simulink model "RecurDyn_Host_Block_23_2"  (R2024a)
settings: Solver=ode45  StartTime=0.0  StopTime=1.0  FixedStep=Control_timestep  RelTol=1e-3  AbsTol=1e-6
values from neighbouring files (symbols this model uses):
  GCoSim_Name = 'GCoSim1'    [car_ver1_GCoSim1.m]    (also in car_ver1_GCoSim2.m = 'GCoSim2'; pure_GCoSim1.m)
  GCoSim_Name_n = r_temp___(2)    [car_ver1_GCoSim1.m]    (also in car_ver1_GCoSim2.m; pure_GCoSim1.m)
  Matlab_version = str2double(splited_Version__(1))    [car_ver1_GCoSim1.m]    (also in car_ver1_GCoSim2.m; pure_GCoSim1.m)
  Output_File = 'car_ver1_GCoSim1_GCoSim1'    [car_ver1_GCoSim1.m]    (also in car_ver1_GCoSim2.m = 'car_ver1_GCoSimulink_GCoSim2'; pure_GCoSim1.m = 'pure_GCoSim1')
  Output_file_n = r_temp___(2)    [car_ver1_GCoSim1.m]    (also in car_ver1_GCoSim2.m; pure_GCoSim1.m)
  Plant_inputs_num = r_temp___(1)    [car_ver1_GCoSim1.m]    (also in car_ver1_GCoSim2.m; pure_GCoSim1.m)
  Plant_outputs_num = r_temp___(1)    [car_ver1_GCoSim1.m]    (also in car_ver1_GCoSim2.m; pure_GCoSim1.m)
  RecurDyn = 'C:\Program Files\FunctionBay, Inc\RecurDyn 2024\Bin\'    [car_ver1_GCoSim1.m]    (also in car_ver1_GCoSim2.m; pure_GCoSim1.m)
  RecurDyn_controltimestep = 1.e-003    (= 0.001)    [car_ver1_GCoSim1.m]    (also in car_ver1_GCoSim2.m; pure_GCoSim1.m)
  RecurDyn_model = 'car_ver1.rdyn'    [car_ver1_GCoSim1.m]    (also in car_ver1_GCoSim2.m; pure_GCoSim1.m = 'pure.rdyn')
  RecurDyn_model_n = r_temp___(2)    [car_ver1_GCoSim1.m]    (also in car_ver1_GCoSim2.m; pure_GCoSim1.m)
settings Model: Creator=hgildong  LastModifiedBy=Dell
settings SolverCC: AutoScaleAbsTol=off  AlgebraicLoopSolver=TrustRegion
settings DataIOCC: SaveFormat=Array  SignalLoggingSaveFormat=ModelDataLogs  ReturnWorkspaceOutputs=off
settings OptimizationCC: BooleanDataType=off  ExpressionDepthLimit=2147483647  InitFltsAndDblsToZero=on  LifeSpan=inf
settings DebuggingCC: SaveWithParameterizedLinksMsg=none  UnderspecifiedInitializationDetection=Classic  MergeDetectMultiDrivingBlocksExec=none  SignalResolutionControl=TryResolveAllWithWarning  MultiTaskDSMMsg=warning  MultiTaskCondExecSysMsg=none  FcnCallInpInsideContextMsg=warning  UnconnectedInputMsg=warning  UnconnectedOutputMsg=warning  UnconnectedLineMsg=warning  StateNameClashWarn=warning  SFUnexpectedBacktrackingDiag=warning  SFNoUnconditionalDefaultTransitionDiag=warning  SFExecutionAtInitializationDiag=none  ArithmeticOperatorsInVariantConditions=warning
settings HardwareCC: ProdBitPerPointer=32  ProdBitPerSizeT=32  ProdBitPerPtrDiffT=32  ProdLargestAtomicFloat=None  ProdIntDivRoundTo=Undefined  ProdEndianess=Unspecified  ProdWordSize=32  ProdHWDeviceType=32-bit Generic  TargetUnknown=on
settings ModelReferenceCC: EnableRefExpFcnMdlSchedulingChecks=on  PropagateSignalLabelsOutOfModel=off
settings SFSimCC: SimUseLocalCustomCode=off  CustomCodeUndefinedFunction=UseInterfaceOnly
settings RTWCC: TemplateMakefile=grt_unix.tmf  RTWUseLocalCustomCode=off  GPUComputeCapability=3.5
settings CodeAppCC: StateflowObjectComments=on
settings GRTTargetCC: TargetFcnLib=ansi_tfl_tmw.mat  TargetLangStandard=C89/C90 (ANSI)  ModelReferenceCompliant=off  CombineOutputUpdateFcns=off  MatFileLogging=off  GRTInterface=on
settings ConfigComp: CovMetricSettings=dw  CovSaveCumulativeToWorkspaceVar=on  CovSaveSingleToWorkspaceVar=on  CovExternalEMLEnable=off

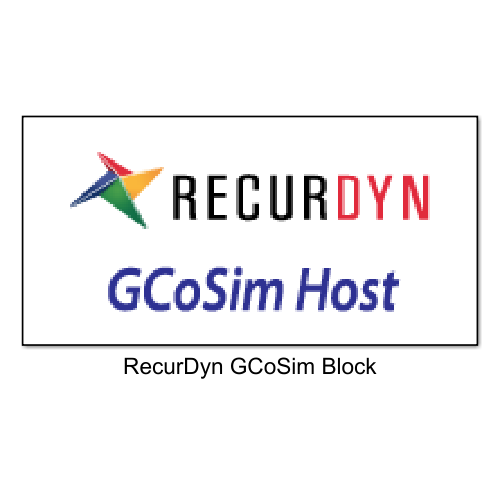
[thumbnail: Simulink's stored preview of the top-level diagram]
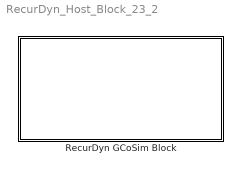
== system RecurDyn_Host_Block_23_2 ==
  RecurDyn GCoSim Block : Subsystem
      mask Display: image(imread('RecurDyn_GCoSimIF_Host.png'))

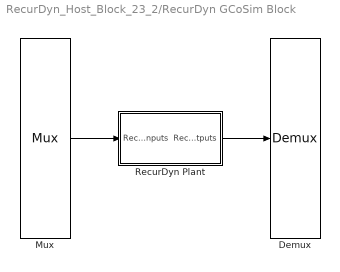
== system RecurDyn_Host_Block_23_2/RecurDyn GCoSim Block ==
  Demux : Demux  Outputs=1
      settings: DisplayOption=none
  Mux : Mux  Inputs=1
  RecurDyn Plant : Subsystem  mask(Recurdyn/Plant){RecurDyn_model_name=RecurDyn_model, GCoSim_Name_=GCoSim_Name, Output_File_Name_=Output_File, RecurDyn_=RecurDyn, Matlab_version_=Matlab_version, RecurDyn_controltimestep_=RecurDyn_controltimestep, RecurDyn_step_=100, Waitingtime=1000, RecurDyn_static_=off, RecurDyn_show_=on, RecurDyn_ani_=on, Create_Output_Folder_=off}
      mask prompts: GCoSim_Name_ "GCoSim Name"; Output_File_Name_ "Output File Name"; RecurDyn_ "RecurDyn_install_directory"; Matlab_version_ "Matlab version"; RecurDyn_controltimestep_ "Sampling period"; RecurDyn_step_ "RecurDyn_step"; Waitingtime "Waiting time"; RecurDyn_static_ "Static analysis"; RecurDyn_show_ "RecurDyn_show"; RecurDyn_ani_ "RecurDyn_animation"; Create_Output_Folder_ "Create Output Folder"
      mask help:
      | This block is able to simulate for any Recurdyn Dynamics Model as Recurdyn/GCoSim Solver.
      | All Data of Plant inputs/outputs are transfered at every sampling time which is defined by Sampling Period (Control Time Step).
      mask Display: disp( 'Dynamic Model' )
  wires:
  RecurDyn Plant/1(RecurDyn_outputs) -> Demux/1
  Mux/1 -> RecurDyn Plant/1(" RecurDyn_inputs")

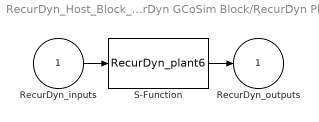
== system RecurDyn_Host_Block_23_2/RecurDyn GCoSim Block/RecurDyn Plant ==
  " RecurDyn_inputs" : Inport
  S-Function : S-Function  FunctionName=RecurDyn_plant6  Parameters=RecurDyn_controltimestep_,RecurDyn_model_name,RecurDyn_,RecurDyn_static_,RecurDyn_step_,RecurDyn_show_,RecurDyn_ani_,Matlab_version_,RecurDyn_model_n,Plant_inputs_num,Plant_outputs_num,Waitingtime,Create_Output_Folder_,Output_File_Name_,Output_file_n,GCoSim_Name_,GCoSim_Name_n  SFunctionDeploymentMode=off  EnableBusSupport=off
  RecurDyn_outputs : Outport  InitialOutput=0  VectorParamsAs1DForOutWhenUnconnected=off
  wires:
  S-Function/1 -> RecurDyn_outputs/1
  " RecurDyn_inputs"/1 -> S-Function/1
